simulink model "W01_current"  (R2024b)
settings: Solver=ode4  StartTime=0  StopTime=T_final  FixedStep=h  RelTol=1e-3
StopFcn:
  | W01_cur_plot;
values from neighbouring files (symbols this model uses):
  animate = 1    [W01_0_setup.m]    (also in W01_setup.m)
  beta_c = 0    [W01_0_setup.m]    (also in W01_setup.m)
  h = 0.02    [W01_0_setup.m]    (also in W01_1_build_openloop.m = Simulink.Annotation([m '/note']); W01_E_build_current.m = Simulink.Annotation([sub '/note']); W01_F_build_interactive.m = Simulink.Annotation([m '/note']); W01_G_build_rc.m = Simulink.Annotation([m '/note']))
  mp = 25    [W01_0_setup.m]    (also in W01_setup.m)
  n0 = 60    [W01_0_setup.m]    (also in W01_F_button_check.m = str2double(get_param([m '/Drive command/n0'], 'Value')); W01_setup.m)
  rp = [0.05 0 -0.35]'    [W01_0_setup.m]    (also in W01_setup.m)
  V_c = 0    [W01_0_setup.m]    (also in W01_setup.m)
  x0 = zeros(12,1)    [W01_0_setup.m]    (also in W01_E_current_run.m = L0(1) + 16; W01_setup.m)
settings Model: Creator=admin  LastModifiedBy=admin
settings DataIOCC: ReturnWorkspaceOutputs=off

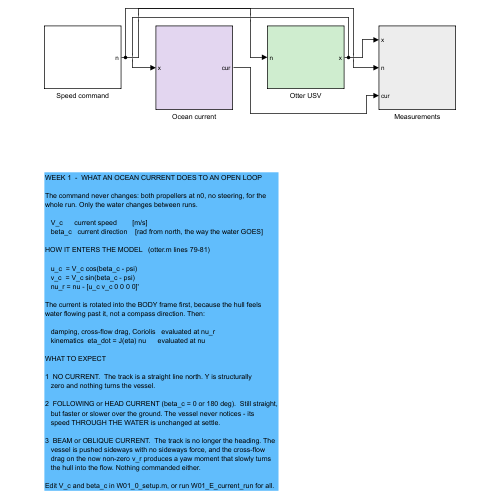
[thumbnail: Simulink's stored preview of the top-level diagram]
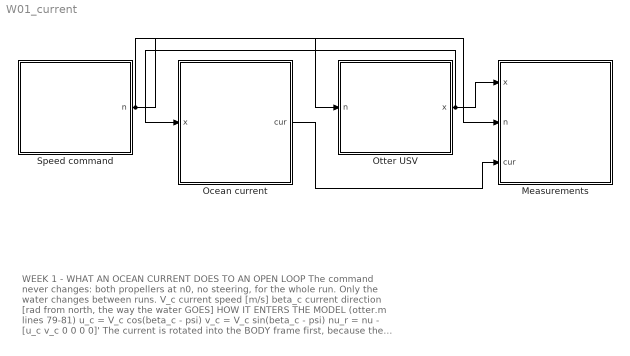
== system W01_current ==
  note: WEEK 1  -  WHAT AN OCEAN CURRENT DOES TO AN OPEN LOOP
      |
      | The command never changes: both propellers at n0, no steering, for the
      | whole run. Only the water changes between runs.
      |
      |    V_c      current speed        [m/s]
      |    beta_c   current direction    [rad from north, the way the water GOES]
      |
      | HOW IT ENTERS THE MODEL   (otter.m lines 79-81)
      |
      |    u_c  = V_c cos(beta_c - psi)
      |    v_c  = V_c sin(beta_c - psi)
      |    nu_r = nu - [u_c v_c 0 0 0 0]'
      |
      | The current is rotated into the BODY frame first, because the hull feels
      | water flowing past it, not a compass direction. Then:
      |
      |    damping, cross-flow drag, Coriolis   evaluated at nu_r
      |    kinematics  eta_dot = J(eta) nu      evaluated at nu
      |
      | WHAT TO EXPECT
      |
      | 1  NO CURRENT.  The track is a straight line north. Y is structurally
      |    zero and nothing turns the vessel.
      |
      | 2  FOLLOWING or HEAD CURRENT (beta_c = 0 or 180 deg).  Still straight,
      |    but faster or slower over the ground. The vessel never notices - its
      |    speed THROUGH THE WATER is unchanged at settle.
      |
      | 3  BEAM or OBLIQUE CURRENT.  The track is no longer the heading. The
      |    vessel is pushed sideways with no sideways force, and the cross-flow
      |    drag on the now non-zero v_r produces a yaw moment that slowly turns
      |    the hull into the flow. Nothing commanded either.
      |
      | Edit V_c and beta_c in W01_0_setup.m, or run W01_E_current_run for all.
  Measurements : Subsystem
  Ocean current : Subsystem
  Otter USV : Subsystem
  Speed command : Subsystem
  wires:
  Speed command/1(n) -> Otter USV/1(n), Measurements/2(n)
  Otter USV/1(x) -> Measurements/1(x), Ocean current/1(x)
  Ocean current/1(cur) -> Measurements/3(cur)

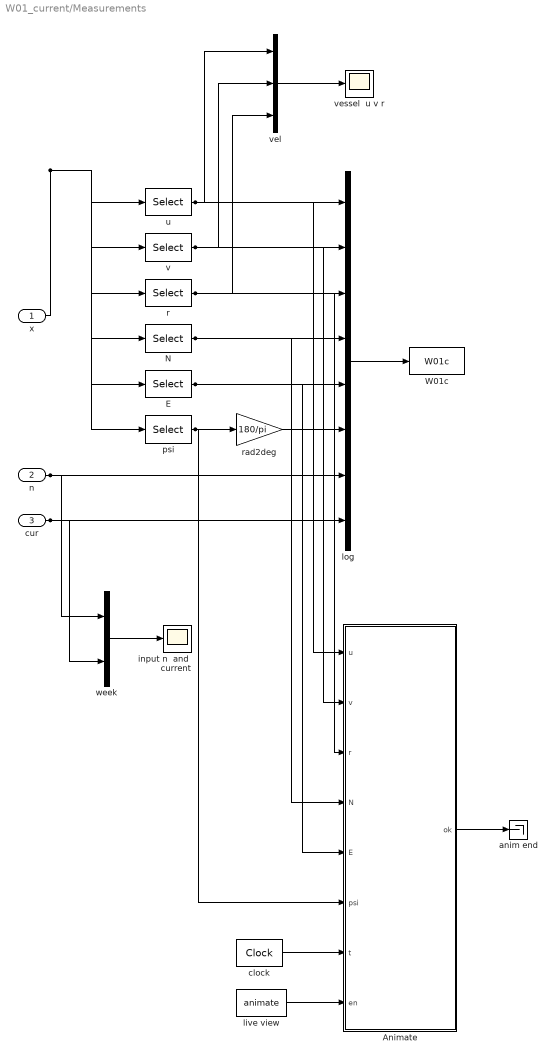
== system W01_current/Measurements ==
  x : Inport
  n : Inport  Port=2
  cur : Inport  Port=3
  Animate : MATLAB Function  TreatAsAtomicUnit=on
  E : Selector  InputPortWidth=12  IndexOptions=Index vector (dialog)  Indices=8  OutputSizes=1
  N : Selector  InputPortWidth=12  IndexOptions=Index vector (dialog)  Indices=7  OutputSizes=1
  W01c : ToWorkspace  VariableName=W01c  SaveFormat=Structure With Time  SampleTime=-1
  anim end : Terminator
  clock : DigitalClock  SampleTime=h
  input n  and  current : Scope
  live view : Constant  Value=animate
  log : Mux  Inputs=8
  psi : Selector  InputPortWidth=12  IndexOptions=Index vector (dialog)  Indices=12  OutputSizes=1
  r : Selector  InputPortWidth=12  IndexOptions=Index vector (dialog)  Indices=6  OutputSizes=1
  rad2deg : Gain  Gain=180/pi
  u : Selector  InputPortWidth=12  IndexOptions=Index vector (dialog)  Indices=1  OutputSizes=1
  v : Selector  InputPortWidth=12  IndexOptions=Index vector (dialog)  Indices=2  OutputSizes=1
  vel : Mux  Inputs=3
  vessel  u v r : Scope
  week : Mux  Inputs=2
  wires:
  x/1 -> u/1, v/1, r/1, N/1, E/1, psi/1
  log/1 -> W01c/1
  psi/1 -> rad2deg/1, Animate/6(psi)
  u/1 -> log/1, vel/1, Animate/1(u)
  v/1 -> log/2, vel/2, Animate/2(v)
  r/1 -> log/3, vel/3, Animate/3(r)
  N/1 -> log/4, Animate/4(N)
  E/1 -> log/5, Animate/5(E)
  rad2deg/1 -> log/6
  n/1 -> log/7, week/1
  cur/1 -> log/8, week/2
  vel/1 -> vessel  u v r/1
  week/1 -> input n  and  current/1
  clock/1 -> Animate/7(t)
  live view/1 -> Animate/8(en)
  Animate/1(ok) -> anim end/1

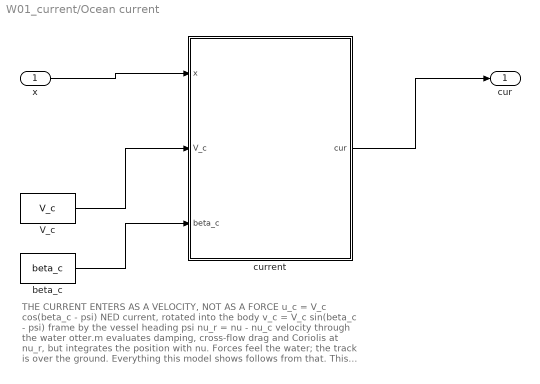
== system W01_current/Ocean current ==
  note: THE CURRENT ENTERS AS A VELOCITY, NOT AS A FORCE
      |
      |    u_c = V_c cos(beta_c - psi)      NED current, rotated into the body
      |    v_c = V_c sin(beta_c - psi)      frame by the vessel heading psi
      |    nu_r = nu - nu_c                 velocity through the water
      |
      | otter.m evaluates damping, cross-flow drag and Coriolis at nu_r, but
      | integrates the position with nu. Forces feel the water; the track is
      | over the ground. Everything this model shows follows from that.
      |
      | This stage drives nothing. It recomputes what the plant already does
      | so that u_r and v_r can be plotted.
  x : Inport
  V_c : Constant  Value=V_c
  beta_c : Constant  Value=beta_c
  current : MATLAB Function  TreatAsAtomicUnit=on
  cur : Outport
  wires:
  x/1 -> current/1(x)
  V_c/1 -> current/2(V_c)
  beta_c/1 -> current/3(beta_c)
  current/1(cur) -> cur/1

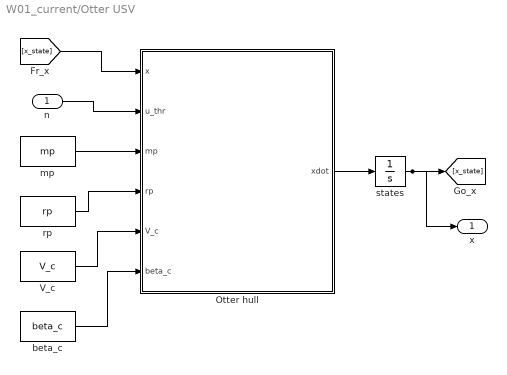
== system W01_current/Otter USV ==
  n : Inport
  Otter hull : MATLAB Function  TreatAsAtomicUnit=on
  V_c : Constant  Value=V_c
  beta_c : Constant  Value=beta_c
  mp : Constant  Value=mp
  rp : Constant  Value=rp
  states : Integrator  InitialCondition=x0
  x : Outport
  wires:
  states/1 -> [x_state], x/1
  [x_state] -> Otter hull/1(x)
  beta_c/1 -> Otter hull/6(beta_c)
  V_c/1 -> Otter hull/5(V_c)
  rp/1 -> Otter hull/4(rp)
  mp/1 -> Otter hull/3(mp)
  n/1 -> Otter hull/2(u_thr)
  Otter hull/1(xdot) -> states/1

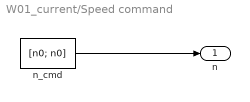
== system W01_current/Speed command ==
  n_cmd : Constant  Value=[n0; n0]
  n : Outport
  wires:
  n_cmd/1 -> n/1

== matlab function W01_current/Otter USV/Otter hull ==
  data: x input; xdot output double size=[12 1]; u_thr input; mp input; rp input; V_c input; beta_c input
function xdot = otter_hull(x, u_thr, mp, rp, V_c, beta_c)
% Fossen's otter.m, called unchanged from Tools/MSS/VESSELS.
%
%   x       12 states, fed back from the integrator
%   u_thr   propeller shaft speeds [rad/s]
%
% otter.m is not written for code generation, so the call is extrinsic and
% xdot has to be pre-sized for Simulink to know the output width.
coder.extrinsic('otter');

xdot = zeros(12,1);
xdot = otter(x, u_thr, mp, rp, V_c, beta_c);
end

== matlab function W01_current/Ocean current/current ==
  data: x input; cur output double size=[4 1]; V_c input; beta_c input
function cur = current(x, V_c, beta_c)
%#codegen
%CURRENT  The two lines otter.m runs on its lines 79-81, made visible.
%
%  A current is given in NED by a speed and a direction. The hull does not
%  feel NED; it feels water flowing past it. So the current is rotated into
%  the body frame by the vessel's own heading before it is subtracted.
%
%    u_c = V_c cos(beta_c - psi)
%    v_c = V_c sin(beta_c - psi)
%
%  beta_c is the direction the water FLOWS TOWARDS, measured from north.
%  With beta_c = 0 the water sets north; a vessel heading north then has a
%  FOLLOWING current and meets less resistance.
%
%  nu_r is what every hydrodynamic term in otter.m is evaluated at. nu is
%  what the kinematics integrates. The gap between them is the drift.
psi = x(12);
u   = x(1);
v   = x(2);

u_c = V_c * cos(beta_c - psi);
v_c = V_c * sin(beta_c - psi);

u_r = u - u_c;
v_r = v - v_c;

cur = [u_c; v_c; u_r; v_r];

== matlab function W01_current/Measurements/Animate ==
  data: u input; ok output; v input; r input; N input; E input; psi input; t input; en input
function ok = Animate(u, v, r, N, E, psi, t, en)
%#codegen
% Live view of the vessel while the model runs.
%
% A MATLAB Function block cannot plot, so the drawing function is declared
% extrinsic: Simulink calls plain MATLAB rather than generating code for it.
% Set animate = 0 in the setup script to switch the live view off.
%
% psi arrives in RADIANS and r in rad/s - the units otter.m works in. The
% wrapper converts them for display, in one place, so no two figures in the
% course can disagree about what a degree is.
coder.extrinsic('W01c_animate');
ok = 1;
if en > 0.5
    W01c_animate(u, v, r, N, E, psi, t);
end
end
